simulink model "Modelo_del_sistema"  (R2018a)
settings: Solver=VariableStepAuto  StartTime=0  StopTime=2678400  FixedStep=45  RelTol=1e-3  EnableMultiTasking=on
libraries: simulink x2
(part 1 of 2)
settings Model: Creator=»Paul117x«  LastModifiedBy=Paul
settings OptimizationCC: LifeSpan=inf
settings DebuggingCC: SFUnexpectedBacktrackingDiag=warning  SFNoUnconditionalDefaultTransitionDiag=warning  SFExecutionAtInitializationDiag=none
settings CodeAppCC: StateflowObjectComments=on
settings GRTTargetCC: TargetLangStandard=C89/C90 (ANSI)  GeneratePreprocessorConditionals=Disable all
settings ConfigComp: CovMetricSettings=dw  CovHtmlReporting=on  CovSaveCumulativeToWorkspaceVar=on  CovSaveSingleToWorkspaceVar=on  CovExternalEMLEnable=off
settings SimscapeCC: SimscapeNormalizeSystem=off

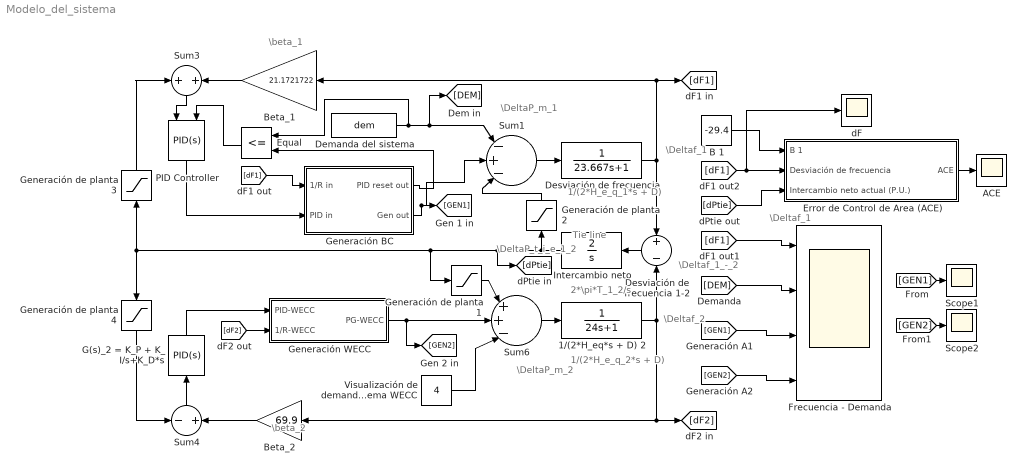
== system Modelo_del_sistema ==
  note: \Deltaf_1
  note: 2*\pi*T_1_2/s
  note: 1/(2*H_e_q_1*s + D)
  note: \beta_2
  note: \beta_1
  note: Tie line
  note: \DeltaP_m_2
  note: \Deltaf_1_-_2
  note: \DeltaP_t_i_e_1_2
  note: \Deltaf_2
  note: \Deltaf_1
  note: \DeltaP_m_1
  note: 1/(2*H_e_q_2*s + D)
  1/(2*H_eq*s + D) 2 : TransferFcn  Denominator=[24 1]
  ACE : Scope
  B 1 : Constant  Value=-29.4
  Beta_1 : Gain  Gain=21.1721722
  Beta_2 : Gain  Gain=69.9
  Demanda del sistema : FromWorkspace  VariableName=dem  SampleTime=0
  Desviación de frecuencia : TransferFcn  Denominator=[23.667 1]
  Desviación de frecuencia 1-2 : Sum  Inputs=+|-
  Equal : RelationalOperator  Operator=<=  OutDataTypeStr=boolean  RndMeth=Simplest
  Error de Control de Area (ACE) : Subsystem
  Frecuencia - Demanda : Scope  NumInputPorts=4
  G(s)_2 = K_P + K_I/s+K_D*s : simulink/Continuous/PID Controller  Controller=PID  TimeDomain=Continuous-time  SampleTime=-1  IntegratorMethod=Forward Euler  FilterMethod=Forward Euler  Form=Parallel  UseFilter=on  ControllerParametersSource=internal  P=0  I=0.00249882658784488  D=0  N=100  InitialConditionSource=internal  InitialConditionForIntegrator=0  InitialConditionForFilter=0  ExternalReset=none  LimitOutput=off  UpperSaturationLimit=inf  LowerSaturationLimit=-inf  LinearizeAsGain=on  AntiWindupMode=none  Kb=1  TrackingMode=off  Kt=1  PParamMin=[]  PParamMax=[]  IParamMin=[]  IParamMax=[]  DParamMin=[]  DParamMax=[]  NParamMin=[]  NParamMax=[]  KbParamMin=[]  KbParamMax=[]  KtParamMin=[]  KtParamMax=[]  POutMin=[]  POutMax=[]  IOutMin=[]  IOutMax=[]  DOutMin=[]  DOutMax=[]  NOutMin=[]  NOutMax=[]  KbOutMin=[]  KbOutMax=[]  KtOutMin=[]  KtOutMax=[]  IntegratorOutMin=[]  IntegratorOutMax=[]  FilterOutMin=[]  FilterOutMax=[]  SumOutMin=[]  SumOutMax=[]  SumI1OutMin=[]  SumI1OutMax=[]  SumI2OutMin=[]  SumI2OutMax=[]  SumI3OutMin=[]  SumI3OutMax=[]  SumDOutMin=[]  SumDOutMax=[]  SaturationOutMin=[]  SaturationOutMax=[]  IntegratorContinuousStateAttributes=''  IntegratorStateMustResolveToSignalObject=off  IntegratorRTWStateStorageClass=Auto  FilterContinuousStateAttributes=''  FilterStateMustResolveToSignalObject=off  FilterRTWStateStorageClass=Auto  DifferentiatorICPrevScaledInput=0  DifferentiatorOutMin=[]  DifferentiatorOutMax=[]  FilterDiffOutCoefMin=[]  FilterDiffOutCoefMax=[]  SumDenOutMin=[]  SumDenOutMax=[]  SumNumOutMin=[]  SumNumOutMax=[]  ReciprocalOutMin=[]  ReciprocalOutMax=[]  DivideOutMin=[]  DivideOutMax=[]  TunerSelectOption=Transfer Function Based (PID Tuner App)
  Generación BC : Subsystem
  Generación WECC : Subsystem
  Generación de planta 1 : Saturate  UpperLimit=0.4  LowerLimit=-0.8
  Generación de planta 2 : Saturate  UpperLimit=0.8  LowerLimit=-0.4
  Generación de planta 3 : Saturate  UpperLimit=0.8  LowerLimit=-0.4
  Generación de planta 4 : Saturate  UpperLimit=0.4  LowerLimit=-0.8
  Intercambio neto : TransferFcn  Numerator=[2]  Denominator=[1 0]
  PID Controller : simulink/Continuous/PID Controller  Controller=PID  TimeDomain=Continuous-time  SampleTime=-1  IntegratorMethod=Forward Euler  FilterMethod=Forward Euler  Form=Parallel  UseFilter=on  ControllerParametersSource=internal  P=0  I=0.00419020704903793  D=0  N=100  InitialConditionSource=internal  InitialConditionForIntegrator=0  InitialConditionForFilter=0  ExternalReset=falling  LimitOutput=on  UpperSaturationLimit=2.577  LowerSaturationLimit=-2.577  LinearizeAsGain=on  AntiWindupMode=clamping  Kb=1  TrackingMode=off  Kt=1  PParamMin=[]  PParamMax=[]  IParamMin=[]  IParamMax=[]  DParamMin=[]  DParamMax=[]  NParamMin=[]  NParamMax=[]  KbParamMin=[]  KbParamMax=[]  KtParamMin=[]  KtParamMax=[]  POutMin=[]  POutMax=[]  IOutMin=[]  IOutMax=[]  DOutMin=[]  DOutMax=[]  NOutMin=[]  NOutMax=[]  KbOutMin=[]  KbOutMax=[]  KtOutMin=[]  KtOutMax=[]  IntegratorOutMin=[]  IntegratorOutMax=[]  FilterOutMin=[]  FilterOutMax=[]  SumOutMin=[]  SumOutMax=[]  SumI1OutMin=[]  SumI1OutMax=[]  SumI2OutMin=[]  SumI2OutMax=[]  SumI3OutMin=[]  SumI3OutMax=[]  SumDOutMin=[]  SumDOutMax=[]  SaturationOutMin=[]  SaturationOutMax=[]  IntegratorContinuousStateAttributes=''  IntegratorStateMustResolveToSignalObject=off  IntegratorRTWStateStorageClass=Auto  FilterContinuousStateAttributes=''  FilterStateMustResolveToSignalObject=off  FilterRTWStateStorageClass=Auto  DifferentiatorICPrevScaledInput=0  DifferentiatorOutMin=[]  DifferentiatorOutMax=[]  FilterDiffOutCoefMin=[]  FilterDiffOutCoefMax=[]  SumDenOutMin=[]  SumDenOutMax=[]  SumNumOutMin=[]  SumNumOutMax=[]  ReciprocalOutMin=[]  ReciprocalOutMax=[]  DivideOutMin=[]  DivideOutMax=[]  TunerSelectOption=Transfer Function Based (PID Tuner App)
  Scope1 : Scope
  Scope2 : Scope
  Sum1 : Sum  Inputs=||-|+|-||
  Sum3 : Sum  Inputs=+|+
  Sum4 : Sum  Inputs=-|+
  Sum6 : Sum  Inputs=||+|+|-||
  Visualización de demanda en sistema WECC : Constant  Value=4
  dF : Scope
  wires:
  Sum1/1 -> Desviación de frecuencia/1
  1/(2*H_eq*s + D) 2/1 -> Desviación de frecuencia 1-2/2, [dF2], Beta_2/1
  Beta_1/1 -> Sum3/2
  Beta_2/1 -> Sum4/2
  Sum4/1 -> G(s)_2 = K_P + K_I/s+K_D*s/1
  B 1/1 -> Error de Control de Area (ACE)/1(B 1)
  Error de Control de Area (ACE)/1(ACE) -> ACE/1
  G(s)_2 = K_P + K_I/s+K_D*s/1 -> Generación WECC/1(PID-WECC)
  Desviación de frecuencia 1-2/1 -> Intercambio neto/1
  Sum6/1 -> 1/(2*H_eq*s + D) 2/1
  Generación WECC/1(PG-WECC) -> Sum6/2, [GEN2]
  [DEM] -> Frecuencia - Demanda/2
  Demanda del sistema/1 -> Equal/1, Sum1/1, [DEM]
  Visualización de demanda en sistema WECC/1 -> Sum6/3
  Intercambio neto/1 -> Generación de planta 1/1, Generación de planta 4/1, Generación de planta 3/1, [dPtie], Generación de planta 2/1
  Generación de planta 1/1 -> Sum6/1
  Sum3/1 -> PID Controller/1
  PID Controller/1 -> Generación BC/2(PID in)
  Equal/1 -> PID Controller/2
  [dF1] -> Generación BC/1(1/R in)
  Generación BC/1(PID reset out) -> Equal/2
  Generación BC/2(Gen out) -> Sum1/2, [GEN1]
  [dF1] -> Frecuencia - Demanda/1
  [dF2] -> Generación WECC/2(1/R-WECC)
  [dPtie] -> Error de Control de Area (ACE)/3(Intercambio neto actual (P.U.))
  Desviación de frecuencia/1 -> [dF1], Beta_1/1, Desviación de frecuencia 1-2/1
  [GEN2] -> Frecuencia - Demanda/4
  [GEN1] -> Frecuencia - Demanda/3
  [dF1] -> dF/1, Error de Control de Area (ACE)/2(Desviación de frecuencia)
  [GEN1] -> Scope1/1
  [GEN2] -> Scope2/1
  Generación de planta 2/1 -> Sum1/3
  Generación de planta 3/1 -> Sum3/1
  Generación de planta 4/1 -> Sum4/1

== system Modelo_del_sistema/Error de Control de Area (ACE) ==
  note: \Deltaf_1
  note: Conversión de frecuencia
      | 	     P.U. a Hz.
  note: 10*B_i*(\Deltaf)
  note: IN_a - IN_p
  note: Conversión de intercambio
      | 	     P.U. a MW.
  B 1 : Inport
  Desviación de frecuencia : Inport  Port=2
  Intercambio neto actual (P.U.) : Inport  Port=3
  Constante : Constant  Value=10
  Hz Base : Constant  Value=60
  Intercambio programado (MW) : Constant  Value=0
  MW Base : Constant  Value=1000
  Product{,1..3} (4 alike) : Product  Inputs=**
  Sum7 : Sum  Inputs=+|-
  Sum9 : Sum  Inputs=-|+
  ACE : Outport
  wires:
  B 1/1 -> Product2/2
  Hz Base/1 -> Product/2
  Product/1 -> Product1/1
  MW Base/1 -> Product3/2
  Sum9/1 -> ACE/1
  Constante/1 -> Product1/2
  Product2/1 -> Sum9/1
  Sum7/1 -> Sum9/2
  Desviación de frecuencia/1 -> Product/1
  Intercambio neto actual (P.U.)/1 -> Product3/1
  Product3/1 -> Sum7/1
  Intercambio programado (MW)/1 -> Sum7/2
  Product1/1 -> Product2/1

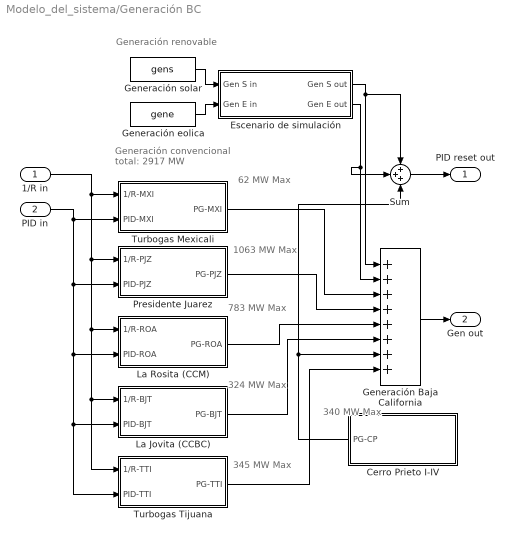
== system Modelo_del_sistema/Generación BC ==
  note: Generación renovable
  note: Generación convencional
      | 	 total: 2917 MW
  note: 62 MW
      |   Max
  note: 1063 MW
      |     Max
  note: 783 MW
      |    Max
  note: 324 MW
      |    Max
  note: 340 MW
      |   Max
  note: 345 MW
      |    Max
  1/R in : Inport
  PID in : Inport  Port=2
  Cerro Prieto I-IV : Subsystem
  Escenario de simulación : Subsystem
  Generación Baja California : Sum  Inputs=+||+||+||+||+||+||+||+
  Generación eolica : FromWorkspace  VariableName=gene  SampleTime=0
  Generación solar : FromWorkspace  VariableName=gens  SampleTime=0
  La Jovita (CCBC) : Subsystem
  La Rosita (CCM) : Subsystem
  Presidente Juarez : Subsystem
  Sum : Sum  Inputs=3
  Turbogas Mexicali : Subsystem
  Turbogas Tijuana : Subsystem
  PID reset out : Outport
  Gen out : Outport  Port=2
  wires:
  La Jovita (CCBC)/1(PG-BJT) -> Generación Baja California/6
  Generación solar/1 -> Escenario de simulación/1(Gen S in)
  PID in/1 -> Turbogas Mexicali/2(PID-MXI), Presidente Juarez/2(PID-PJZ), La Rosita (CCM)/2(PID-ROA), La Jovita (CCBC)/2(PID-BJT), Turbogas Tijuana/2(PID-TTI)
  Escenario de simulación/2(Gen E out) -> Sum/2, Generación Baja California/2
  1/R in/1 -> Turbogas Mexicali/1(1/R-MXI), Presidente Juarez/1(1/R-PJZ), La Rosita (CCM)/1(1/R-ROA), La Jovita (CCBC)/1(1/R-BJT), Turbogas Tijuana/1(1/R-TTI)
  Escenario de simulación/1(Gen S out) -> Sum/1, Generación Baja California/1
  Cerro Prieto I-IV/1(PG-CP) -> Sum/3, Generación Baja California/7
  Presidente Juarez/1(PG-PJZ) -> Generación Baja California/4
  Generación eolica/1 -> Escenario de simulación/2(Gen E in)
  Turbogas Mexicali/1(PG-MXI) -> Generación Baja California/3
  Turbogas Tijuana/1(PG-TTI) -> Generación Baja California/8
  Generación Baja California/1 -> Gen out/1
  La Rosita (CCM)/1(PG-ROA) -> Generación Baja California/5
  Sum/1 -> PID reset out/1

== system Modelo_del_sistema/Generación WECC ==
  PID-WECC : Inport
  1/R-WECC : Inport  Port=2
  1/(sT_g + 1) 2 : TransferFcn  Denominator=[0.04 1]
  1/R2 : Gain  Gain=20
  Generación extra área 2 : TransferFcn  Denominator=[0.2 1]
  Sum5 : Sum  Inputs=|--
  PG-WECC : Outport
  wires:
  1/R2/1 -> Sum5/2
  PID-WECC/1 -> Sum5/1
  1/R-WECC/1 -> 1/R2/1
  1/(sT_g + 1) 2/1 -> Generación extra área 2/1
  Sum5/1 -> 1/(sT_g + 1) 2/1
  Generación extra área 2/1 -> PG-WECC/1

== system Modelo_del_sistema/Generación BC/Cerro Prieto I-IV ==
  note: Heq = 4.593
  CP Gen : Constant  Value=0.34
  PG-CP : Outport
  wires:
  CP Gen/1 -> PG-CP/1

== system Modelo_del_sistema/Generación BC/Escenario de simulación ==
  Gen S in : Inport
  Gen E in : Inport  Port=2
  Constant : Constant  Value=0
  Eólico Ago : Subsystem
  Eólico Dic : Subsystem
  Multiport Switch : MultiPortSwitch  Inputs=2  DataPortForDefault=Additional data port
  Multiport Switch2 : MultiPortSwitch  Inputs=2  DataPortForDefault=Additional data port
  Scope : Scope
  Selector : FromWorkspace  VariableName=p  OutDataTypeStr=double  SampleTime=0  OutputAfterFinalValue=Holding final value
  Solar Ago : Subsystem
  Solar Dic : Subsystem
  Gen S out : Outport
  Gen E out : Outport  Port=2
  wires:
  Gen E in/1 -> Eólico Ago/1(Gen E in), Eólico Dic/1(Gen E in)
  Eólico Ago/1(Gen E out) -> Multiport Switch2/2
  Eólico Dic/1(Gen E out) -> Multiport Switch2/3
  Multiport Switch2/1 -> Scope/1, Gen E out/1
  Multiport Switch/1 -> Gen S out/1
  Selector/1 -> Multiport Switch/1, Multiport Switch2/1
  Constant/1 -> Multiport Switch2/4, Multiport Switch/4
  Solar Dic/1(Gen S out) -> Multiport Switch/3
  Solar Ago/1(Gen S out) -> Multiport Switch/2
  Gen S in/1 -> Solar Dic/1(Gen S in), Solar Ago/1(Gen S in)

== system Modelo_del_sistema/Generación BC/La Jovita (CCBC) ==
  note: Heq = 4.2
  1/R-BJT : Inport
  PID-BJT : Inport  Port=2
  1/(sT_g + 1)1 : TransferFcn  Denominator=[2.675 1]
  1/(sT_t + 1)1 : TransferFcn  Denominator=[0.71 1]
  1/R2 : Gain  Gain=16.50615303
  Saturation : Saturate  UpperLimit=0.324  LowerLimit=0
  Sum1 : Sum  Inputs=--|
  PG-BJT : Outport
  wires:
  1/(sT_g + 1)1/1 -> 1/(sT_t + 1)1/1
  Sum1/1 -> 1/(sT_g + 1)1/1
  1/R-BJT/1 -> 1/R2/1
  1/R2/1 -> Sum1/1
  1/(sT_t + 1)1/1 -> Saturation/1
  Saturation/1 -> PG-BJT/1
  PID-BJT/1 -> Sum1/2

== system Modelo_del_sistema/Generación BC/La Rosita (CCM) ==
  note: T2 = 0.2
  note: 1/R = 24.85720114
  note: T_1 = 1
  note: Heq = 5.893
  1/R-ROA : Inport
  PID-ROA : Inport  Port=2
  1/(sT_g + 1)1 : TransferFcn  Denominator=[0.15 1]
  1/(sT_t + 1)1 : TransferFcn  Denominator=[0.05 1]
  1/R1 : Gain  Gain=24.85720114
  Saturation : Saturate  UpperLimit=0.783  LowerLimit=0
  Sum1 : Sum  Inputs=--|
  PG-ROA : Outport
  wires:
  1/(sT_g + 1)1/1 -> 1/(sT_t + 1)1/1
  Sum1/1 -> 1/(sT_g + 1)1/1
  1/R-ROA/1 -> 1/R1/1
  1/R1/1 -> Sum1/1
  1/(sT_t + 1)1/1 -> Saturation/1
  Saturation/1 -> PG-ROA/1
  PID-ROA/1 -> Sum1/2

== system Modelo_del_sistema/Generación BC/Presidente Juarez ==
  note: T2 = 1.56
  note: T1 = 2.032
  note: Heq = 3.38
  1/R-PJZ : Inport
  PID-PJZ : Inport  Port=2
  1/(sT_g + 1)1 : TransferFcn  Denominator=[0.2 1]
  1/(sT_t + 1)1 : TransferFcn  Denominator=[0.1 1]
  1/R1 : Gain  Gain=18.56344588
  Saturation : Saturate  UpperLimit=1.063  LowerLimit=0
  Sum1 : Sum  Inputs=--|
  PG-PJZ : Outport
  wires:
  1/(sT_g + 1)1/1 -> 1/(sT_t + 1)1/1
  Sum1/1 -> 1/(sT_g + 1)1/1
  1/R1/1 -> Sum1/1
  1/R-PJZ/1 -> 1/R1/1
  1/(sT_t + 1)1/1 -> Saturation/1
  Saturation/1 -> PG-PJZ/1
  PID-PJZ/1 -> Sum1/2

== system Modelo_del_sistema/Generación BC/Turbogas Mexicali ==
  note: 62 MW de generación MAX
  note: Heq = 3.666
  1/R-MXI : Inport
  PID-MXI : Inport  Port=2
  1/(sT_g + 1) : TransferFcn  Denominator=[0.16666 1]
  1/(sT_t + 1) : TransferFcn  Denominator=[0.366666 1]
  1/R1 : Gain  Gain=19.09999982
  Saturation : Saturate  UpperLimit=0.062  LowerLimit=0
  Sum : Sum  Inputs=--|
  PG-MXI : Outport
  wires:
  1/(sT_g + 1)/1 -> 1/(sT_t + 1)/1
  Sum/1 -> 1/(sT_g + 1)/1
  1/R-MXI/1 -> 1/R1/1
  1/R1/1 -> Sum/1
  1/(sT_t + 1)/1 -> Saturation/1
  Saturation/1 -> PG-MXI/1
  PID-MXI/1 -> Sum/2

== system Modelo_del_sistema/Generación BC/Turbogas Tijuana ==
  note: Heq = 5.91
  1/R-TTI : Inport
  PID-TTI : Inport  Port=2
  1/(sT_g + 1)1 : TransferFcn  Denominator=[0.1 1]
  1/(sT_t + 1)1 : TransferFcn  Denominator=[0.2 1]
  1/R1 : Gain  Gain=21.83406114
  Saturation : Saturate  UpperLimit=0.345  LowerLimit=0
  Sum1 : Sum  Inputs=--|
  PG-TTI : Outport
  wires:
  1/(sT_g + 1)1/1 -> 1/(sT_t + 1)1/1
  Sum1/1 -> 1/(sT_g + 1)1/1
  1/R1/1 -> Sum1/1
  1/R-TTI/1 -> 1/R1/1
  1/(sT_t + 1)1/1 -> Saturation/1
  Saturation/1 -> PG-TTI/1
  PID-TTI/1 -> Sum1/2

== system Modelo_del_sistema/Generación BC/Escenario de simulación/Eólico Ago ==
  Gen E in : Inport
  Falla día 13 : Subsystem
  Falla día 16 : Subsystem
  Falla día 18 : Subsystem
  Falla día 21 : Subsystem
  Falla día 25 : Subsystem
  Falla día 28 : Subsystem
  Falla día 30 : Subsystem
  Falla día 6 : Subsystem
  Falla día 8 : Subsystem
  Gen E out : Outport
  wires:
  Gen E in/1 -> Falla día 6/1(In1)
  Falla día 16/1(Out1) -> Falla día 18/1(In1)
  Falla día 25/1(Out1) -> Falla día 28/1(In1)
  Falla día 28/1(Out1) -> Falla día 30/1(In1)
  Falla día 13/1(Out1) -> Falla día 16/1(In1)
  Falla día 21/1(Out1) -> Falla día 25/1(In1)
  Falla día 30/1(Out1) -> Gen E out/1
  Falla día 18/1(Out1) -> Falla día 21/1(In1)
  Falla día 8/1(Out1) -> Falla día 13/1(In1)
  Falla día 6/1(Out1) -> Falla día 8/1(In1)

== system Modelo_del_sistema/Generación BC/Escenario de simulación/Eólico Dic ==
  Gen E in : Inport
  Falla día 12 : Subsystem
  Falla día 14 : Subsystem
  Falla día 16 : Subsystem
  Falla día 20 : Subsystem
  Falla día 24 : Subsystem
  Falla día 30 : Subsystem
  Falla día 4 : Subsystem
  Falla día 8 : Subsystem
  Falla día 9 : Subsystem
  Gen E out : Outport
  wires:
  Gen E in/1 -> Falla día 4/1(In1)
  Falla día 4/1(Out1) -> Falla día 8/1(In1)
  Falla día 8/1(Out1) -> Falla día 9/1(In1)
  Falla día 9/1(Out1) -> Falla día 12/1(In1)
  Falla día 12/1(Out1) -> Falla día 14/1(In1)
  Falla día 14/1(Out1) -> Falla día 16/1(In1)
  Falla día 16/1(Out1) -> Falla día 20/1(In1)
  Falla día 20/1(Out1) -> Falla día 24/1(In1)
  Falla día 24/1(Out1) -> Falla día 30/1(In1)
  Falla día 30/1(Out1) -> Gen E out/1

== system Modelo_del_sistema/Generación BC/Escenario de simulación/Solar Ago ==
  Gen S in : Inport
  Falla día 12 : Subsystem
  Falla día 16 : Subsystem
  Falla día 18 : Subsystem
  Falla día 20 : Subsystem
  Falla día 25 : Subsystem
  Falla día 26 : Subsystem
  Falla día 28 : Subsystem
  Falla día 5 : Subsystem
  Falla día 9 : Subsystem
  Gen S out : Outport
  wires:
  Falla día 5/1(Out1) -> Falla día 9/1(In1)
  Falla día 9/1(Out1) -> Falla día 12/1(In1)
  Gen S in/1 -> Falla día 5/1(In1)
  Falla día 20/1(Out1) -> Falla día 25/1(In1)
  Falla día 25/1(Out1) -> Falla día 26/1(In1)
  Falla día 26/1(Out1) -> Falla día 28/1(In1)
  Falla día 12/1(Out1) -> Falla día 16/1(In1)
  Falla día 28/1(Out1) -> Gen S out/1
  Falla día 18/1(Out1) -> Falla día 20/1(In1)
  Falla día 16/1(Out1) -> Falla día 18/1(In1)

== system Modelo_del_sistema/Generación BC/Escenario de simulación/Solar Dic ==
  Gen S in : Inport
  Falla día 13 : Subsystem
  Falla día 16 : Subsystem
  Falla día 2 : Subsystem
  Falla día 21 : Subsystem
  Falla día 23 : Subsystem
  Falla día 24 : Subsystem
  Falla día 28 : Subsystem
  Falla día 30 : Subsystem
  Falla día 4 : Subsystem
  Gen S out : Outport
  wires:
  Gen S in/1 -> Falla día 2/1(In1)
  Falla día 4/1(Out1) -> Falla día 13/1(In1)
  Falla día 2/1(Out1) -> Falla día 4/1(In1)
  Falla día 13/1(Out1) -> Falla día 16/1(In1)
  Falla día 16/1(Out1) -> Falla día 21/1(In1)
  Falla día 23/1(Out1) -> Falla día 24/1(In1)
  Falla día 21/1(Out1) -> Falla día 23/1(In1)
  Falla día 24/1(Out1) -> Falla día 28/1(In1)
  Falla día 28/1(Out1) -> Falla día 30/1(In1)
  Falla día 30/1(Out1) -> Gen S out/1

== system Modelo_del_sistema/Generación BC/Escenario de simulación/Eólico Ago/Falla día 13 ==
  In1 : Inport
  Add : Sum
  Clock : Clock
  Clock1 : Clock
  Product : Product
  Sine Wave : Sin  Amplitude=0.73  Frequency=0.00086071/2  Phase=pi/2+pi/4.5  SampleTime=0
  Switch : Switch  Threshold=1097000
  Switch1 : Switch  Threshold=1104300
  Out1 : Outport
  wires:
  Add/1 -> Switch/1
  Product/1 -> Add/2
  Clock/1 -> Switch/2
  In1/1 -> Switch/3, Product/1, Add/1, Switch1/1
  Switch1/1 -> Out1/1
  Sine Wave/1 -> Product/2
  Clock1/1 -> Switch1/2
  Switch/1 -> Switch1/3

== system Modelo_del_sistema/Generación BC/Escenario de simulación/Eólico Ago/Falla día 16 ==
  In1 : Inport
  Add : Sum
  Clock : Clock
  Clock1 : Clock
  Product : Product
  Sine Wave : Sin  Amplitude=0.20  Frequency=0.000455303  Phase=3*pi/2+pi+pi/8.1  SampleTime=0
  Switch : Switch  Threshold=1355000
  Switch1 : Switch  Threshold=1361900
  Out1 : Outport
  wires:
  Add/1 -> Switch/1
  Product/1 -> Add/2
  Clock/1 -> Switch/2
  In1/1 -> Switch/3, Product/1, Add/1, Switch1/1
  Switch1/1 -> Out1/1
  Sine Wave/1 -> Product/2
  Clock1/1 -> Switch1/2
  Switch/1 -> Switch1/3

== system Modelo_del_sistema/Generación BC/Escenario de simulación/Eólico Ago/Falla día 18 ==
  In1 : Inport
  Add : Sum
  Clock : Clock
  Clock1 : Clock
  Product : Product
  Sine Wave : Sin  Amplitude=0.71  Frequency=0.000263999  Phase=pi/4+pi/93  SampleTime=0
  Switch : Switch  Threshold=1532000
  Switch1 : Switch  Threshold=1543900
  Out1 : Outport
  wires:
  Add/1 -> Switch/1
  Product/1 -> Add/2
  Clock/1 -> Switch/2
  In1/1 -> Switch/3, Product/1, Add/1, Switch1/1
  Switch1/1 -> Out1/1
  Sine Wave/1 -> Product/2
  Clock1/1 -> Switch1/2
  Switch/1 -> Switch1/3

== system Modelo_del_sistema/Generación BC/Escenario de simulación/Eólico Ago/Falla día 21 ==
  In1 : Inport
  Add : Sum
  Clock : Clock
  Clock1 : Clock
  Product : Product
  Sine Wave : Sin  Amplitude=0.54  Frequency=0.000213714  Phase=-pi/4-pi/16  SampleTime=0
  Switch : Switch  Threshold=1783300
  Switch1 : Switch  Threshold=1798000
  Out1 : Outport
  wires:
  Add/1 -> Switch/1
  Product/1 -> Add/2
  Clock/1 -> Switch/2
  In1/1 -> Switch/3, Product/1, Add/1, Switch1/1
  Switch1/1 -> Out1/1
  Sine Wave/1 -> Product/2
  Clock1/1 -> Switch1/2
  Switch/1 -> Switch1/3

== system Modelo_del_sistema/Generación BC/Escenario de simulación/Eólico Ago/Falla día 25 ==
  In1 : Inport
  Add : Sum
  Clock : Clock
  Clock1 : Clock
  Product : Product
  Sine Wave : Sin  Amplitude=0.44  Frequency=0.000259636  Phase=pi-pi/4.33  SampleTime=0
  Switch : Switch  Threshold=2132400
  Switch1 : Switch  Threshold=2144500
  Out1 : Outport
  wires:
  Add/1 -> Switch/1
  Product/1 -> Add/2
  Clock/1 -> Switch/2
  In1/1 -> Switch/3, Product/1, Add/1, Switch1/1
  Switch1/1 -> Out1/1
  Sine Wave/1 -> Product/2
  Clock1/1 -> Switch1/2
  Switch/1 -> Switch1/3

== system Modelo_del_sistema/Generación BC/Escenario de simulación/Eólico Ago/Falla día 28 ==
  In1 : Inport
  Add : Sum
  Clock : Clock
  Clock1 : Clock
  Product : Product
  Sine Wave : Sin  Amplitude=0.95  Frequency=0.000255414  Phase=-pi/3.001  SampleTime=0
  Switch : Switch  Threshold=2402600
  Switch1 : Switch  Threshold=2414900
  Out1 : Outport
  wires:
  Add/1 -> Switch/1
  Product/1 -> Add/2
  Clock/1 -> Switch/2
  In1/1 -> Switch/3, Product/1, Add/1, Switch1/1
  Switch1/1 -> Out1/1
  Sine Wave/1 -> Product/2
  Clock1/1 -> Switch1/2
  Switch/1 -> Switch1/3

== system Modelo_del_sistema/Generación BC/Escenario de simulación/Eólico Ago/Falla día 30 ==
  In1 : Inport
  Add : Sum
  Clock : Clock
  Clock1 : Clock
  Product : Product
  Sine Wave : Sin  Amplitude=0.93  Frequency=0.000119000  Phase=-pi/32.76  SampleTime=0
  Switch : Switch  Threshold=2561600
  Switch1 : Switch  Threshold=2588000
  Out1 : Outport
  wires:
  Add/1 -> Switch/1
  Product/1 -> Add/2
  Clock/1 -> Switch/2
  In1/1 -> Switch/3, Product/1, Add/1, Switch1/1
  Switch1/1 -> Out1/1
  Sine Wave/1 -> Product/2
  Clock1/1 -> Switch1/2
  Switch/1 -> Switch1/3

== system Modelo_del_sistema/Generación BC/Escenario de simulación/Eólico Ago/Falla día 6 ==
  In1 : Inport
  Add : Sum
  Clock : Clock
  Clock1 : Clock
  Product : Product
  Scope : Scope  NumInputPorts=2
  Sine Wave : Sin  Amplitude=0.52  Frequency=0.000213714  Phase=pi/2+pi+pi/42  SampleTime=0
  Switch : Switch  Threshold=492100
  Switch1 : Switch  Threshold=506800
  Out1 : Outport
  wires:
  Add/1 -> Switch/1
  Product/1 -> Add/2
  Clock/1 -> Switch/2
  In1/1 -> Scope/1, Switch/3, Product/1, Add/1, Switch1/1
  Switch1/1 -> Scope/2, Out1/1
  Sine Wave/1 -> Product/2
  Clock1/1 -> Switch1/2
  Switch/1 -> Switch1/3

== system Modelo_del_sistema/Generación BC/Escenario de simulación/Eólico Ago/Falla día 8 ==
  In1 : Inport
  Add : Sum
  Clock : Clock
  Clock1 : Clock
  Product : Product
  Sine Wave : Sin  Amplitude=0.62  Frequency=3.779359583e-4/2  Phase=-pi/2-pi/24  SampleTime=0
  Switch : Switch  Threshold=657450
  Switch1 : Switch  Threshold=674075
  Out1 : Outport
  wires:
  Add/1 -> Switch/1
  Product/1 -> Add/2
  Clock/1 -> Switch/2
  In1/1 -> Switch/3, Product/1, Add/1, Switch1/1
  Switch1/1 -> Out1/1
  Sine Wave/1 -> Product/2
  Clock1/1 -> Switch1/2
  Switch/1 -> Switch1/3

== system Modelo_del_sistema/Generación BC/Escenario de simulación/Eólico Dic/Falla día 12 ==
  In1 : Inport
  Add : Sum
  Clock : Clock
  Clock1 : Clock
  Product : Product
  Sine Wave : Sin  Amplitude=0.94  Frequency=0.000475999  Phase=pi-pi/3.66  SampleTime=0
  Switch : Switch  Threshold=991800
  Switch1 : Switch  Threshold=998400
  Out1 : Outport
  wires:
  Add/1 -> Switch/1
  Product/1 -> Add/2
  Clock/1 -> Switch/2
  In1/1 -> Product/1, Add/1, Switch1/1, Switch/3
  Switch1/1 -> Out1/1
  Sine Wave/1 -> Product/2
  Clock1/1 -> Switch1/2
  Switch/1 -> Switch1/3

== system Modelo_del_sistema/Generación BC/Escenario de simulación/Eólico Dic/Falla día 14 ==
  In1 : Inport
  Add : Sum
  Clock : Clock
  Clock1 : Clock
  Product : Product
  Sine Wave : Sin  Amplitude=0.20  Frequency=0.000180551  Phase=-3*pi/4-pi/23.5  SampleTime=0
  Switch : Switch  Threshold=1179600
  Switch1 : Switch  Threshold=1197000
  Out1 : Outport
  wires:
  Add/1 -> Switch/1
  Product/1 -> Add/2
  Clock/1 -> Switch/2
  In1/1 -> Product/1, Add/1, Switch1/1, Switch/3
  Switch1/1 -> Out1/1
  Sine Wave/1 -> Product/2
  Clock1/1 -> Switch1/2
  Switch/1 -> Switch1/3

== system Modelo_del_sistema/Generación BC/Escenario de simulación/Eólico Dic/Falla día 16 ==
  In1 : Inport
  Add : Sum
  Clock : Clock
  Clock1 : Clock
  Product : Product
  Sine Wave : Sin  Amplitude=0.41  Frequency=0.000515015  Phase=-pi/2-pi/128  SampleTime=0
  Switch : Switch  Threshold=1326800
  Switch1 : Switch  Threshold=1332900
  Out1 : Outport
  wires:
  Add/1 -> Switch/1
  Product/1 -> Add/2
  Clock/1 -> Switch/2
  In1/1 -> Switch/3, Product/1, Add/1, Switch1/1
  Switch1/1 -> Out1/1
  Sine Wave/1 -> Product/2
  Clock1/1 -> Switch1/2
  Switch/1 -> Switch1/3

== system Modelo_del_sistema/Generación BC/Escenario de simulación/Eólico Dic/Falla día 20 ==
  In1 : Inport
  Add : Sum
  Clock : Clock
  Clock1 : Clock
  Product : Product
  Sine Wave : Sin  Amplitude=0.36  Frequency=0.000356999  Phase=-pi/2-pi/10  SampleTime=0
  Switch : Switch  Threshold=1686100
  Switch1 : Switch  Threshold=1694900
  Out1 : Outport
  wires:
  Add/1 -> Switch/1
  Product/1 -> Add/2
  Clock/1 -> Switch/2
  In1/1 -> Switch/3, Product/1, Add/1, Switch1/1
  Switch1/1 -> Out1/1
  Sine Wave/1 -> Product/2
  Clock1/1 -> Switch1/2
  Switch/1 -> Switch1/3

== system Modelo_del_sistema/Generación BC/Escenario de simulación/Eólico Dic/Falla día 24 ==
  In1 : Inport
  Add : Sum
  Clock : Clock
  Clock1 : Clock
  Product : Product
  Sine Wave : Sin  Amplitude=0.59  Frequency=0.000345230  Phase=pi-pi/10.1  SampleTime=0
  Switch : Switch  Threshold=2002900
  Switch1 : Switch  Threshold=2012000
  Out1 : Outport
  wires:
  Add/1 -> Switch/1
  Product/1 -> Add/2
  Clock/1 -> Switch/2
  In1/1 -> Switch/3, Product/1, Add/1, Switch1/1
  Switch1/1 -> Out1/1
  Sine Wave/1 -> Product/2
  Clock1/1 -> Switch1/2
  Switch/1 -> Switch1/3

== system Modelo_del_sistema/Generación BC/Escenario de simulación/Eólico Dic/Falla día 30 ==
  In1 : Inport
  Add : Sum
  Clock : Clock
  Clock1 : Clock
  Product : Product
  Sine Wave : Sin  Amplitude=0.3  Frequency=0.000073060  Phase=pi/2+pi/10.21  SampleTime=0
  Switch : Switch  Threshold=2511300
  Switch1 : Switch  Threshold=2554300
  Out1 : Outport
  wires:
  Add/1 -> Switch/1
  Product/1 -> Add/2
  Clock/1 -> Switch/2
  In1/1 -> Switch/3, Product/1, Add/1, Switch1/1
  Switch1/1 -> Out1/1
  Sine Wave/1 -> Product/2
  Clock1/1 -> Switch1/2
  Switch/1 -> Switch1/3

== system Modelo_del_sistema/Generación BC/Escenario de simulación/Eólico Dic/Falla día 4 ==
  In1 : Inport
  Add : Sum
  Clock : Clock
  Clock1 : Clock
  Product : Product
  Sine Wave : Sin  Amplitude=0.6  Frequency=2.992e-4  Phase=-pi/2-pi/4-pi/46.5  SampleTime=0
  Switch : Switch  Threshold=312600
  Switch1 : Switch  Threshold=323100
  Out1 : Outport
  wires:
  Add/1 -> Switch/1
  Product/1 -> Add/2
  Clock/1 -> Switch/2
  In1/1 -> Switch/3, Product/1, Add/1, Switch1/1
  Switch1/1 -> Out1/1
  Sine Wave/1 -> Product/2
  Clock1/1 -> Switch1/2
  Switch/1 -> Switch1/3

== system Modelo_del_sistema/Generación BC/Escenario de simulación/Eólico Dic/Falla día 8 ==
  In1 : Inport
  Add : Sum
  Clock : Clock
  Clock1 : Clock
  Product : Product
  Sine Wave : Sin  Amplitude=0.41  Frequency=0.000951998  Phase=-pi/1.57  SampleTime=0
  Switch : Switch  Threshold=632400
  Switch1 : Switch  Threshold=635700
  Out1 : Outport
  wires:
  Add/1 -> Switch/1
  Product/1 -> Add/2
  Clock/1 -> Switch/2
  In1/1 -> Switch/3, Product/1, Add/1, Switch1/1
  Switch1/1 -> Out1/1
  Sine Wave/1 -> Product/2
  Clock1/1 -> Switch1/2
  Switch/1 -> Switch1/3

== system Modelo_del_sistema/Generación BC/Escenario de simulación/Eólico Dic/Falla día 9 ==
  In1 : Inport
  Add : Sum
  Clock : Clock
  Clock1 : Clock
  Product : Product
  Sine Wave : Sin  Amplitude=0.21  Frequency=0.000448799  Phase=-pi-pi/3.69  SampleTime=0
  Switch : Switch  Threshold=743900
  Switch1 : Switch  Threshold=750900
  Out1 : Outport
  wires:
  Add/1 -> Switch/1
  Product/1 -> Add/2
  Clock/1 -> Switch/2
  In1/1 -> Product/1, Add/1, Switch1/1, Switch/3
  Switch1/1 -> Out1/1
  Sine Wave/1 -> Product/2
  Clock1/1 -> Switch1/2
  Switch/1 -> Switch1/3

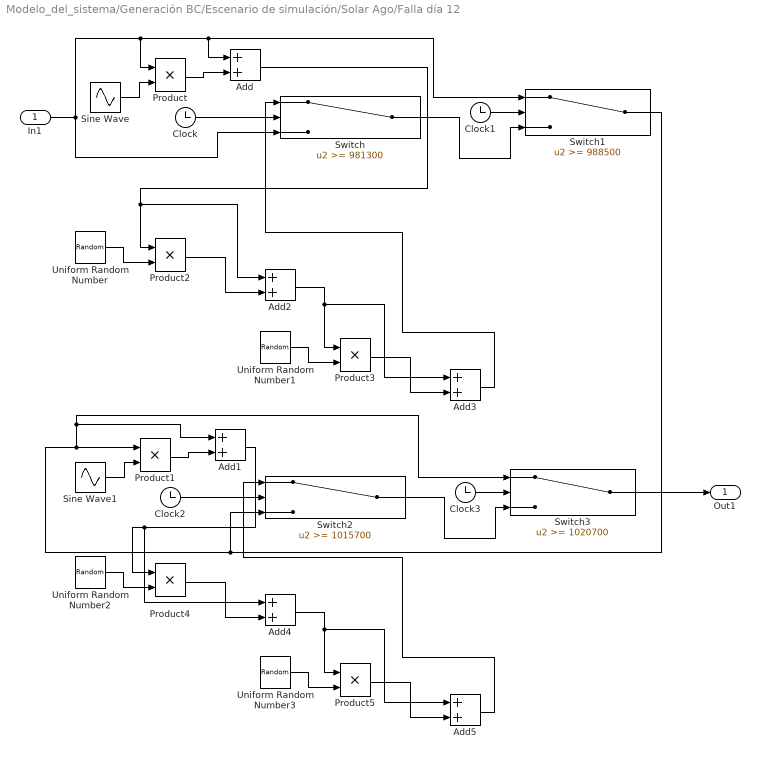
== system Modelo_del_sistema/Generación BC/Escenario de simulación/Solar Ago/Falla día 12 ==
  In1 : Inport
  Add{,1..5} (6 alike) : Sum
  Clock{,1..3} (4 alike) : Clock
  Product{,1..5} (6 alike) : Product
  Sine Wave : Sin  Amplitude=0.27  Frequency=0.000436332  Phase=pi-pi/3.4299  SampleTime=0
  Sine Wave1 : Sin  Amplitude=0.56  Frequency=0.000628319  Phase=-pi/8-pi/67  SampleTime=0
  Switch : Switch  Threshold=981300
  Switch1 : Switch  Threshold=988500
  Switch2 : Switch  Threshold=1015700
  Switch3 : Switch  Threshold=1020700
  Uniform Random Number : UniformRandomNumber  Minimum=-0.5  Maximum=0  Seed=1337  SampleTime=50
  Uniform Random Number1 : UniformRandomNumber  Minimum=-0.25  Maximum=0  Seed=69420  SampleTime=25
  Uniform Random Number2 : UniformRandomNumber  Minimum=-0.5  Maximum=0  Seed=1337  SampleTime=50
  Uniform Random Number3 : UniformRandomNumber  Minimum=-0.25  Maximum=0  Seed=69420  SampleTime=25
  Out1 : Outport
  wires:
  Product/1 -> Add/2
  Clock/1 -> Switch/2
  Sine Wave/1 -> Product/2
  Clock1/1 -> Switch1/2
  Switch/1 -> Switch1/3
  In1/1 -> Switch/3, Product/1, Add/1, Switch1/1
  Product1/1 -> Add1/2
  Clock2/1 -> Switch2/2
  Sine Wave1/1 -> Product1/2
  Clock3/1 -> Switch3/2
  Switch2/1 -> Switch3/3
  Switch3/1 -> Out1/1
  Switch1/1 -> Switch3/1, Add1/1, Product1/1, Switch2/3
  Add2/1 -> Add3/1, Product3/1
  Product3/1 -> Add3/2
  Add3/1 -> Switch/1
  Uniform Random Number1/1 -> Product3/2
  Add/1 -> Add2/1, Product2/1
  Uniform Random Number/1 -> Product2/2
  Product2/1 -> Add2/2
  Add4/1 -> Add5/1, Product5/1
  Product5/1 -> Add5/2
  Add5/1 -> Switch2/1
  Uniform Random Number3/1 -> Product5/2
  Add1/1 -> Add4/1, Product4/1
  Uniform Random Number2/1 -> Product4/2
  Product4/1 -> Add4/2

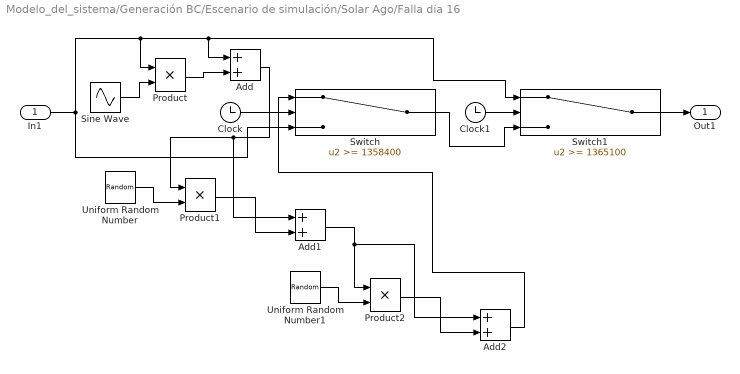
== system Modelo_del_sistema/Generación BC/Escenario de simulación/Solar Ago/Falla día 16 ==
  In1 : Inport
  Add : Sum
  Add1 : Sum
  Add2 : Sum
  Clock : Clock
  Clock1 : Clock
  Product : Product
  Product1 : Product
  Product2 : Product
  Sine Wave : Sin  Amplitude=0.70  Frequency=0.000468894  Phase=-pi/2-pi/6+pi-pi/12.6  SampleTime=0
  Switch : Switch  Threshold=1358400
  Switch1 : Switch  Threshold=1365100
  Uniform Random Number : UniformRandomNumber  Minimum=-0.5  Maximum=0  Seed=1337  SampleTime=50
  Uniform Random Number1 : UniformRandomNumber  Minimum=-0.25  Maximum=0  Seed=69420  SampleTime=25
  Out1 : Outport
  wires:
  Product/1 -> Add/2
  Clock/1 -> Switch/2
  In1/1 -> Switch/3, Product/1, Add/1, Switch1/1
  Switch1/1 -> Out1/1
  Sine Wave/1 -> Product/2
  Clock1/1 -> Switch1/2
  Switch/1 -> Switch1/3
  Add1/1 -> Add2/1, Product2/1
  Product2/1 -> Add2/2
  Add2/1 -> Switch/1
  Uniform Random Number1/1 -> Product2/2
  Add/1 -> Add1/1, Product1/1
  Uniform Random Number/1 -> Product1/2
  Product1/1 -> Add1/2

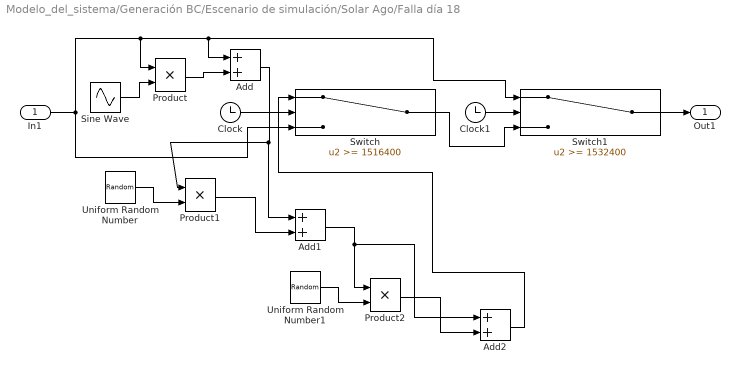
== system Modelo_del_sistema/Generación BC/Escenario de simulación/Solar Ago/Falla día 18 ==
  In1 : Inport
  Add : Sum
  Add1 : Sum
  Add2 : Sum
  Clock : Clock
  Clock1 : Clock
  Product : Product
  Product1 : Product
  Product2 : Product
  Sine Wave : Sin  Amplitude=0.29  Frequency=0.000196350  Phase=pi/4-pi/40  SampleTime=0
  Switch : Switch  Threshold=1516400
  Switch1 : Switch  Threshold=1532400
  Uniform Random Number : UniformRandomNumber  Minimum=-0.5  Maximum=0  Seed=1337  SampleTime=50
  Uniform Random Number1 : UniformRandomNumber  Minimum=-0.25  Maximum=0  Seed=69420  SampleTime=25
  Out1 : Outport
  wires:
  Product/1 -> Add/2
  Clock/1 -> Switch/2
  In1/1 -> Switch/3, Product/1, Add/1, Switch1/1
  Switch1/1 -> Out1/1
  Sine Wave/1 -> Product/2
  Clock1/1 -> Switch1/2
  Switch/1 -> Switch1/3
  Add1/1 -> Add2/1, Product2/1
  Add/1 -> Add1/1, Product1/1
  Product2/1 -> Add2/2
  Add2/1 -> Switch/1
  Uniform Random Number1/1 -> Product2/2
  Uniform Random Number/1 -> Product1/2
  Product1/1 -> Add1/2

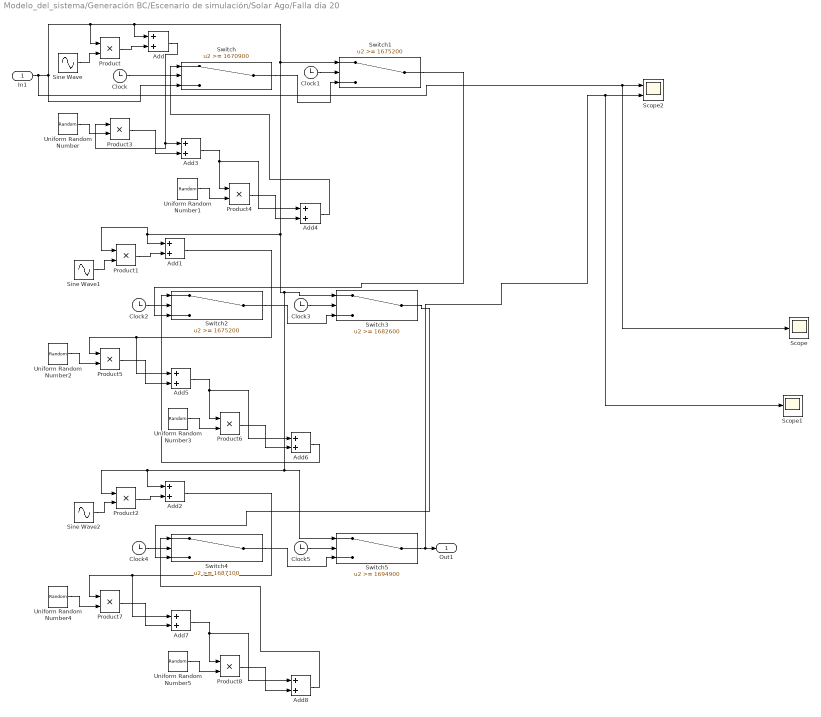
== system Modelo_del_sistema/Generación BC/Escenario de simulación/Solar Ago/Falla día 20 ==
  In1 : Inport
  Add{,1..8} (9 alike) : Sum
  Clock{,1..5} (6 alike) : Clock
  Product{,1..8} (9 alike) : Product
  Scope : Scope
  Scope1 : Scope
  Scope2 : Scope  NumInputPorts=2
  Sine Wave : Sin  Amplitude=0.57  Frequency=1.461206e-3/2  Phase=pi/2-pi/12  SampleTime=0
  Sine Wave1 : Sin  Amplitude=0.92  Frequency=8.49079e-4/2  Phase=pi-pi/2.65  SampleTime=0
  Sine Wave2 : Sin  Amplitude=0.33  Frequency=8.05537e-4/2  Phase=pi-pi/3.4  SampleTime=0
  Switch : Switch  Threshold=1670900
  Switch1 : Switch  Threshold=1675200
  Switch2 : Switch  Threshold=1675200
  Switch3 : Switch  Threshold=1682600
  Switch4 : Switch  Threshold=1687100
  Switch5 : Switch  Threshold=1694900
  Uniform Random Number : UniformRandomNumber  Minimum=-0.5  Maximum=0  Seed=1337  SampleTime=50
  Uniform Random Number1 : UniformRandomNumber  Minimum=-0.25  Maximum=0  Seed=69420  SampleTime=25
  Uniform Random Number2 : UniformRandomNumber  Minimum=-0.5  Maximum=0  Seed=1337  SampleTime=50
  Uniform Random Number3 : UniformRandomNumber  Minimum=-0.25  Maximum=0  Seed=69420  SampleTime=25
  Uniform Random Number4 : UniformRandomNumber  Minimum=-0.5  Maximum=0  Seed=1337  SampleTime=50
  Uniform Random Number5 : UniformRandomNumber  Minimum=-0.25  Maximum=0  Seed=69420  SampleTime=25
  Out1 : Outport
  wires:
  Product/1 -> Add/2
  Clock/1 -> Switch/2
  Sine Wave/1 -> Product/2
  Clock1/1 -> Switch1/2
  Switch/1 -> Switch1/3
  Switch1/1 -> Switch2/3
  Switch2/1 -> Switch3/3
  Clock2/1 -> Switch2/2
  Clock3/1 -> Switch3/2
  Sine Wave1/1 -> Product1/2
  Product1/1 -> Add1/2
  In1/1 -> Scope/1, Scope2/1, Switch/3, Product/1, Add/1, Switch1/1, Product2/1, Add2/1, Switch5/1, Switch3/1, Product1/1, Add1/1
  Switch3/1 -> Switch4/3
  Switch4/1 -> Switch5/3
  Clock4/1 -> Switch4/2
  Clock5/1 -> Switch5/2
  Sine Wave2/1 -> Product2/2
  Product2/1 -> Add2/2
  Switch5/1 -> Out1/1, Scope1/1, Scope2/2
  Add3/1 -> Add4/1, Product4/1
  Add/1 -> Product3/1, Add3/1
  Product4/1 -> Add4/2
  Add4/1 -> Switch/1
  Uniform Random Number1/1 -> Product4/2
  Uniform Random Number/1 -> Product3/2
  Product3/1 -> Add3/2
  Add5/1 -> Add6/1, Product6/1
  Product6/1 -> Add6/2
  Uniform Random Number3/1 -> Product6/2
  Add1/1 -> Add5/1, Product5/1
  Uniform Random Number2/1 -> Product5/2
  Product5/1 -> Add5/2
  Add6/1 -> Switch2/1
  Add7/1 -> Add8/1, Product8/1
  Product8/1 -> Add8/2
  Add8/1 -> Switch4/1
  Uniform Random Number5/1 -> Product8/2
  Add2/1 -> Add7/1, Product7/1
  Uniform Random Number4/1 -> Product7/2
  Product7/1 -> Add7/2

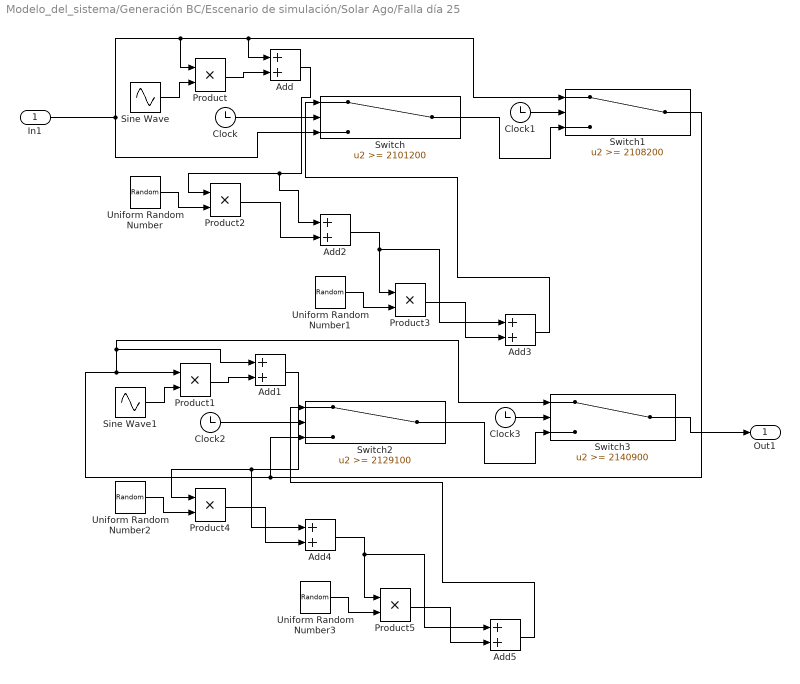
== system Modelo_del_sistema/Generación BC/Escenario de simulación/Solar Ago/Falla día 25 ==
  In1 : Inport
  Add{,1..5} (6 alike) : Sum
  Clock{,1..3} (4 alike) : Clock
  Product{,1..5} (6 alike) : Product
  Sine Wave : Sin  Amplitude=0.62  Frequency=0.000448799  Phase=pi-pi/5.833  SampleTime=0
  Sine Wave1 : Sin  Amplitude=0.66  Frequency=0.000266237  Phase=pi/2+pi/14.798  SampleTime=0
  Switch : Switch  Threshold=2101200
  Switch1 : Switch  Threshold=2108200
  Switch2 : Switch  Threshold=2129100
  Switch3 : Switch  Threshold=2140900
  Uniform Random Number : UniformRandomNumber  Minimum=-0.5  Maximum=0  Seed=1337  SampleTime=50
  Uniform Random Number1 : UniformRandomNumber  Minimum=-0.25  Maximum=0  Seed=69420  SampleTime=25
  Uniform Random Number2 : UniformRandomNumber  Minimum=-0.5  Maximum=0  Seed=1337  SampleTime=50
  Uniform Random Number3 : UniformRandomNumber  Minimum=-0.25  Maximum=0  Seed=69420  SampleTime=25
  Out1 : Outport
  wires:
  Switch3/1 -> Out1/1
  Product/1 -> Add/2
  Clock/1 -> Switch/2
  Sine Wave/1 -> Product/2
  Clock1/1 -> Switch1/2
  Switch/1 -> Switch1/3
  In1/1 -> Switch/3, Product/1, Add/1, Switch1/1
  Product1/1 -> Add1/2
  Clock2/1 -> Switch2/2
  Sine Wave1/1 -> Product1/2
  Clock3/1 -> Switch3/2
  Switch2/1 -> Switch3/3
  Switch1/1 -> Switch3/1, Add1/1, Product1/1, Switch2/3
  Add2/1 -> Add3/1, Product3/1
  Add/1 -> Add2/1, Product2/1
  Product3/1 -> Add3/2
  Add3/1 -> Switch/1
  Uniform Random Number1/1 -> Product3/2
  Uniform Random Number/1 -> Product2/2
  Product2/1 -> Add2/2
  Add4/1 -> Add5/1, Product5/1
  Product5/1 -> Add5/2
  Add5/1 -> Switch2/1
  Uniform Random Number3/1 -> Product5/2
  Add1/1 -> Add4/1, Product4/1
  Uniform Random Number2/1 -> Product4/2
  Product4/1 -> Add4/2

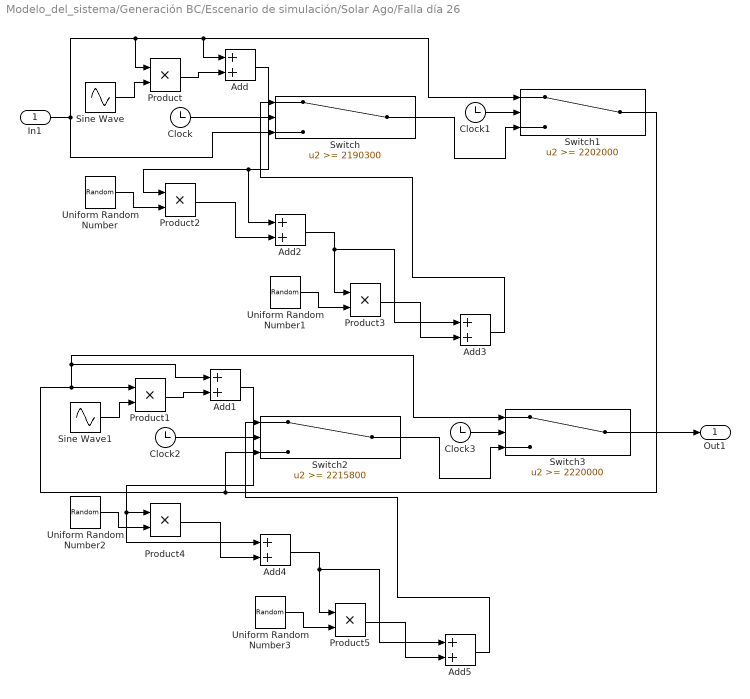
== system Modelo_del_sistema/Generación BC/Escenario de simulación/Solar Ago/Falla día 26 ==
  In1 : Inport
  Add{,1..5} (6 alike) : Sum
  Clock{,1..3} (4 alike) : Clock
  Product{,1..5} (6 alike) : Product
  Sine Wave : Sin  Amplitude=0.79  Frequency=0.000268512  Phase=-pi/4+pi/22.21  SampleTime=0
  Sine Wave1 : Sin  Amplitude=0.39  Frequency=0.000747998  Phase=-pi/2-pi/14.04  SampleTime=0
  Switch : Switch  Threshold=2190300
  Switch1 : Switch  Threshold=2202000
  Switch2 : Switch  Threshold=2215800
  Switch3 : Switch  Threshold=2220000
  Uniform Random Number : UniformRandomNumber  Minimum=-0.5  Maximum=0  Seed=1337  SampleTime=50
  Uniform Random Number1 : UniformRandomNumber  Minimum=-0.25  Maximum=0  Seed=69420  SampleTime=25
  Uniform Random Number2 : UniformRandomNumber  Minimum=-0.5  Maximum=0  Seed=1337  SampleTime=50
  Uniform Random Number3 : UniformRandomNumber  Minimum=-0.25  Maximum=0  Seed=69420  SampleTime=25
  Out1 : Outport
  wires:
  Product/1 -> Add/2
  Clock/1 -> Switch/2
  Sine Wave/1 -> Product/2
  Clock1/1 -> Switch1/2
  Switch/1 -> Switch1/3
  In1/1 -> Switch/3, Product/1, Add/1, Switch1/1
  Product1/1 -> Add1/2
  Clock2/1 -> Switch2/2
  Sine Wave1/1 -> Product1/2
  Clock3/1 -> Switch3/2
  Switch2/1 -> Switch3/3
  Switch3/1 -> Out1/1
  Switch1/1 -> Switch3/1, Add1/1, Product1/1, Switch2/3
  Add2/1 -> Add3/1, Product3/1
  Product3/1 -> Add3/2
  Add3/1 -> Switch/1
  Uniform Random Number1/1 -> Product3/2
  Add/1 -> Add2/1, Product2/1
  Uniform Random Number/1 -> Product2/2
  Product2/1 -> Add2/2
  Add4/1 -> Add5/1, Product5/1
  Product5/1 -> Add5/2
  Add5/1 -> Switch2/1
  Uniform Random Number3/1 -> Product5/2
  Add1/1 -> Add4/1, Product4/1
  Uniform Random Number2/1 -> Product4/2
  Product4/1 -> Add4/2

== system Modelo_del_sistema/Generación BC/Escenario de simulación/Solar Ago/Falla día 28 ==
  In1 : Inport
  Add : Sum
  Add1 : Sum
  Add2 : Sum
  Clock : Clock
  Clock1 : Clock
  Product : Product
  Product1 : Product
  Product2 : Product
  Sine Wave : Sin  Amplitude=0.56  Frequency=2.596358e-3/2  Phase=pi/7.15  SampleTime=0
  Switch : Switch  Threshold=2378520
  Switch1 : Switch  Threshold=2380940
  Uniform Random Number : UniformRandomNumber  Minimum=-0.5  Maximum=0  Seed=1337  SampleTime=50
  Uniform Random Number1 : UniformRandomNumber  Minimum=-0.25  Maximum=0  Seed=69420  SampleTime=25
  Out1 : Outport
  wires:
  Product/1 -> Add/2
  Clock/1 -> Switch/2
  In1/1 -> Switch/3, Product/1, Add/1, Switch1/1
  Switch1/1 -> Out1/1
  Sine Wave/1 -> Product/2
  Clock1/1 -> Switch1/2
  Switch/1 -> Switch1/3
  Add1/1 -> Add2/1, Product2/1
  Product2/1 -> Add2/2
  Add2/1 -> Switch/1
  Uniform Random Number1/1 -> Product2/2
  Add/1 -> Add1/1, Product1/1
  Uniform Random Number/1 -> Product1/2
  Product1/1 -> Add1/2

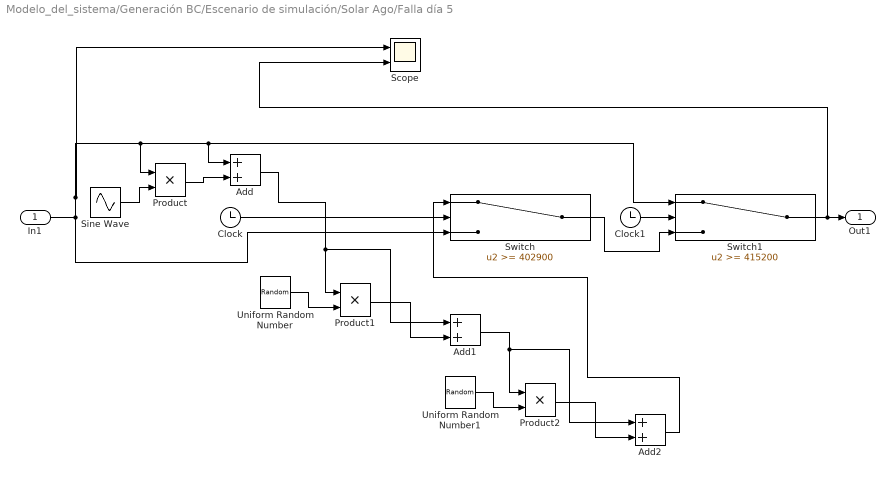
== system Modelo_del_sistema/Generación BC/Escenario de simulación/Solar Ago/Falla día 5 ==
  In1 : Inport
  Add : Sum
  Add1 : Sum
  Add2 : Sum
  Clock : Clock
  Clock1 : Clock
  Product : Product
  Product1 : Product
  Product2 : Product
  Scope : Scope  NumInputPorts=2
  Sine Wave : Sin  Amplitude=0.81  Frequency=0.000255414  Phase=pi/4-pi/165  SampleTime=0
  Switch : Switch  Threshold=402900
  Switch1 : Switch  Threshold=415200
  Uniform Random Number : UniformRandomNumber  Minimum=-0.5  Maximum=0  Seed=1337  SampleTime=50
  Uniform Random Number1 : UniformRandomNumber  Minimum=-0.25  Maximum=0  Seed=69420  SampleTime=25
  Out1 : Outport
  wires:
  Add/1 -> Add1/1, Product1/1
  Product/1 -> Add/2
  Clock/1 -> Switch/2
  Switch1/1 -> Scope/2, Out1/1
  Sine Wave/1 -> Product/2
  Clock1/1 -> Switch1/2
  Switch/1 -> Switch1/3
  In1/1 -> Switch/3, Scope/1, Product/1, Add/1, Switch1/1
  Uniform Random Number/1 -> Product1/2
  Product1/1 -> Add1/2
  Add2/1 -> Switch/1
  Add1/1 -> Add2/1, Product2/1
  Uniform Random Number1/1 -> Product2/2
  Product2/1 -> Add2/2

== system Modelo_del_sistema/Generación BC/Escenario de simulación/Solar Ago/Falla día 9 ==
  In1 : Inport
  Add : Sum
  Add1 : Sum
  Add2 : Sum
  Clock : Clock
  Clock1 : Clock
  Product : Product
  Product1 : Product
  Product2 : Product
  Sine Wave : Sin  Amplitude=0.56  Frequency=0.000171672  Phase=pi+pi/5.9052  SampleTime=0
  Switch : Switch  Threshold=728900
  Switch1 : Switch  Threshold=747200
  Uniform Random Number : UniformRandomNumber  Minimum=-0.5  Maximum=0  Seed=1337  SampleTime=50
  Uniform Random Number1 : UniformRandomNumber  Minimum=-0.25  Maximum=0  Seed=69420  SampleTime=25
  Out1 : Outport
  wires:
  Product/1 -> Add/2
  Clock/1 -> Switch/2
  Sine Wave/1 -> Product/2
  Clock1/1 -> Switch1/2
  Switch/1 -> Switch1/3
  In1/1 -> Switch/3, Product/1, Add/1, Switch1/1
  Switch1/1 -> Out1/1
  Add1/1 -> Add2/1, Product2/1
  Product2/1 -> Add2/2
  Add2/1 -> Switch/1
  Uniform Random Number1/1 -> Product2/2
  Add/1 -> Add1/1, Product1/1
  Uniform Random Number/1 -> Product1/2
  Product1/1 -> Add1/2

== system Modelo_del_sistema/Generación BC/Escenario de simulación/Solar Dic/Falla día 13 ==
  In1 : Inport
  Add : Sum
  Add1 : Sum
  Add2 : Sum
  Clock : Clock
  Clock1 : Clock
  Product : Product
  Product1 : Product
  Product2 : Product
  Sine Wave : Sin  Amplitude=0.31  Frequency=0.000184800  Phase=pi/34  SampleTime=0
  Switch : Switch  Threshold=1070500
  Switch1 : Switch  Threshold=1087500
  Uniform Random Number : UniformRandomNumber  Minimum=-0.5  Maximum=0  Seed=1337  SampleTime=50
  Uniform Random Number1 : UniformRandomNumber  Minimum=-0.25  Maximum=0  Seed=69420  SampleTime=25
  Out1 : Outport
  wires:
  Product/1 -> Add/2
  Clock/1 -> Switch/2
  In1/1 -> Switch/3, Product/1, Add/1, Switch1/1
  Switch1/1 -> Out1/1
  Sine Wave/1 -> Product/2
  Clock1/1 -> Switch1/2
  Switch/1 -> Switch1/3
  Add1/1 -> Add2/1, Product2/1
  Product2/1 -> Add2/2
  Add2/1 -> Switch/1
  Uniform Random Number1/1 -> Product2/2
  Add/1 -> Add1/1, Product1/1
  Uniform Random Number/1 -> Product1/2
  Product1/1 -> Add1/2

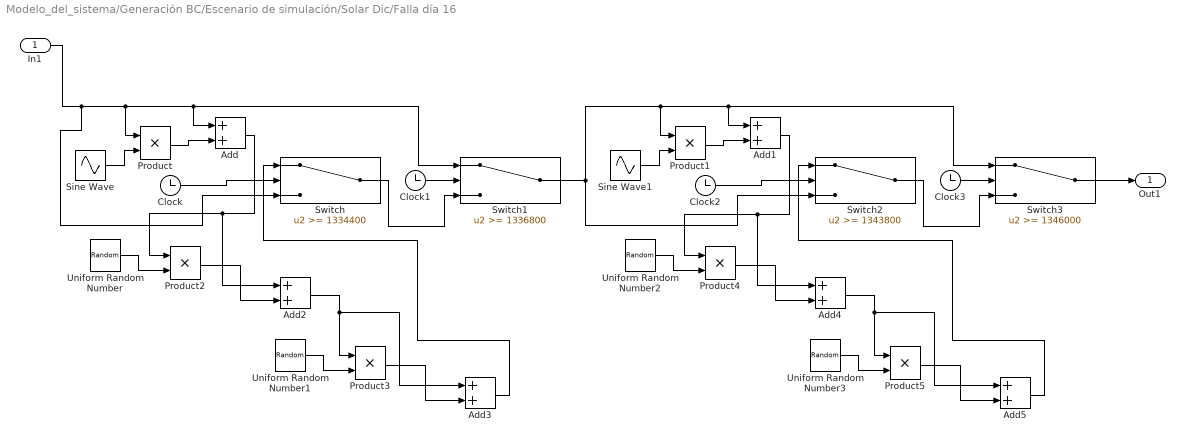
== system Modelo_del_sistema/Generación BC/Escenario de simulación/Solar Dic/Falla día 16 ==
  In1 : Inport
  Add{,1..5} (6 alike) : Sum
  Clock{,1..3} (4 alike) : Clock
  Product{,1..5} (6 alike) : Product
  Sine Wave : Sin  Amplitude=0.57  Frequency=0.001308997  Phase=pi  SampleTime=0
  Sine Wave1 : Sin  Amplitude=0.76  Frequency=0.001427997  Phase=pi/5.5  SampleTime=0
  Switch : Switch  Threshold=1334400
  Switch1 : Switch  Threshold=1336800
  Switch2 : Switch  Threshold=1343800
  Switch3 : Switch  Threshold=1346000
  Uniform Random Number : UniformRandomNumber  Minimum=-0.5  Maximum=0  Seed=1337  SampleTime=50
  Uniform Random Number1 : UniformRandomNumber  Minimum=-0.25  Maximum=0  Seed=69420  SampleTime=25
  Uniform Random Number2 : UniformRandomNumber  Minimum=-0.5  Maximum=0  Seed=1337  SampleTime=50
  Uniform Random Number3 : UniformRandomNumber  Minimum=-0.25  Maximum=0  Seed=69420  SampleTime=25
  Out1 : Outport
  wires:
  Product/1 -> Add/2
  Clock/1 -> Switch/2
  In1/1 -> Switch/3, Product/1, Add/1, Switch1/1
  Sine Wave/1 -> Product/2
  Clock1/1 -> Switch1/2
  Switch/1 -> Switch1/3
  Product1/1 -> Add1/2
  Clock2/1 -> Switch2/2
  Switch1/1 -> Product1/1, Add1/1, Switch3/1, Switch2/3
  Sine Wave1/1 -> Product1/2
  Clock3/1 -> Switch3/2
  Switch2/1 -> Switch3/3
  Switch3/1 -> Out1/1
  Add2/1 -> Add3/1, Product3/1
  Product3/1 -> Add3/2
  Add3/1 -> Switch/1
  Uniform Random Number1/1 -> Product3/2
  Add/1 -> Add2/1, Product2/1
  Uniform Random Number/1 -> Product2/2
  Product2/1 -> Add2/2
  Add4/1 -> Add5/1, Product5/1
  Product5/1 -> Add5/2
  Add5/1 -> Switch2/1
  Uniform Random Number3/1 -> Product5/2
  Add1/1 -> Add4/1, Product4/1
  Uniform Random Number2/1 -> Product4/2
  Product4/1 -> Add4/2

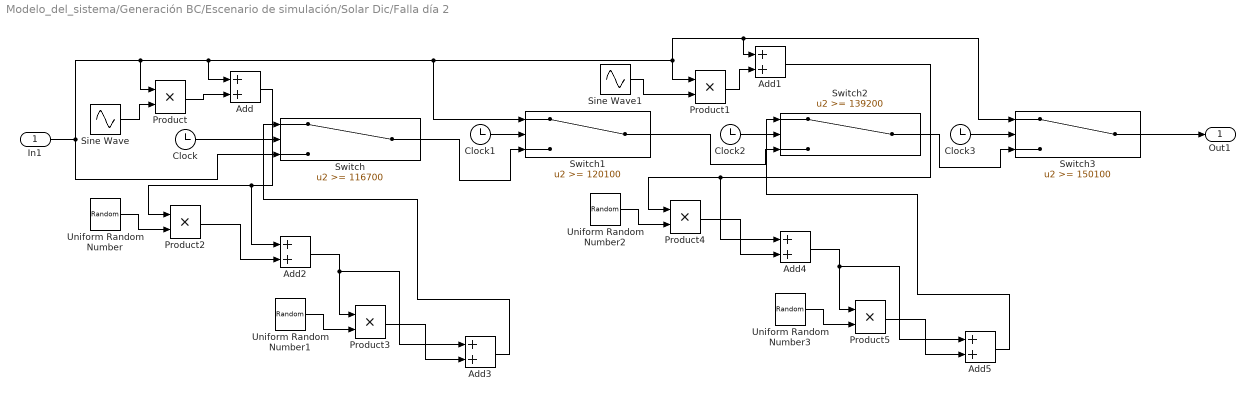
== system Modelo_del_sistema/Generación BC/Escenario de simulación/Solar Dic/Falla día 2 ==
  In1 : Inport
  Add{,1..5} (6 alike) : Sum
  Clock{,1..3} (4 alike) : Clock
  Product{,1..5} (6 alike) : Product
  Sine Wave : Sin  Amplitude=0.63  Frequency=9.23998e-4  Phase=2*pi/4+pi/5.7  SampleTime=0
  Sine Wave1 : Sin  Amplitude=0.82  Frequency=2.88220e-4  Phase=pi/4.36  SampleTime=0
  Switch : Switch  Threshold=116700
  Switch1 : Switch  Threshold=120100
  Switch2 : Switch  Threshold=139200
  Switch3 : Switch  Threshold=150100
  Uniform Random Number : UniformRandomNumber  Minimum=-0.5  Maximum=0  Seed=1337  SampleTime=50
  Uniform Random Number1 : UniformRandomNumber  Minimum=-0.25  Maximum=0  Seed=69420  SampleTime=25
  Uniform Random Number2 : UniformRandomNumber  Minimum=-0.5  Maximum=0  Seed=1337  SampleTime=50
  Uniform Random Number3 : UniformRandomNumber  Minimum=-0.25  Maximum=0  Seed=69420  SampleTime=25
  Out1 : Outport
  wires:
  Product/1 -> Add/2
  Clock/1 -> Switch/2
  Clock1/1 -> Switch1/2
  Switch/1 -> Switch1/3
  Switch1/1 -> Switch2/3
  Switch2/1 -> Switch3/3
  Clock2/1 -> Switch2/2
  Clock3/1 -> Switch3/2
  Sine Wave1/1 -> Product1/2
  Product1/1 -> Add1/2
  In1/1 -> Switch/3, Product/1, Add/1, Switch1/1, Add1/1, Switch3/1, Product1/1
  Sine Wave/1 -> Product/2
  Switch3/1 -> Out1/1
  Add2/1 -> Add3/1, Product3/1
  Product3/1 -> Add3/2
  Uniform Random Number1/1 -> Product3/2
  Add/1 -> Add2/1, Product2/1
  Uniform Random Number/1 -> Product2/2
  Product2/1 -> Add2/2
  Add3/1 -> Switch/1
  Add4/1 -> Add5/1, Product5/1
  Product5/1 -> Add5/2
  Add5/1 -> Switch2/1
  Uniform Random Number3/1 -> Product5/2
  Add1/1 -> Add4/1, Product4/1
  Uniform Random Number2/1 -> Product4/2
  Product4/1 -> Add4/2

== system Modelo_del_sistema/Generación BC/Escenario de simulación/Solar Dic/Falla día 21 ==
  In1 : Inport
  Add : Sum
  Add1 : Sum
  Add2 : Sum
  Clock : Clock
  Clock1 : Clock
  Product : Product
  Product1 : Product
  Product2 : Product
  Sine Wave : Sin  Amplitude=0.43  Frequency=0.000193925  Phase=pi/4+pi/2-pi/111  SampleTime=0
  Switch : Switch  Threshold=1753800
  Switch1 : Switch  Threshold=1770000
  Uniform Random Number : UniformRandomNumber  Minimum=-0.5  Maximum=0  Seed=1337  SampleTime=50
  Uniform Random Number1 : UniformRandomNumber  Minimum=-0.25  Maximum=0  Seed=69420  SampleTime=25
  Out1 : Outport
  wires:
  Product/1 -> Add/2
  Clock/1 -> Switch/2
  In1/1 -> Switch/3, Product/1, Add/1, Switch1/1
  Switch1/1 -> Out1/1
  Sine Wave/1 -> Product/2
  Clock1/1 -> Switch1/2
  Switch/1 -> Switch1/3
  Add1/1 -> Add2/1, Product2/1
  Product2/1 -> Add2/2
  Add2/1 -> Switch/1
  Uniform Random Number1/1 -> Product2/2
  Add/1 -> Add1/1, Product1/1
  Uniform Random Number/1 -> Product1/2
  Product1/1 -> Add1/2

== system Modelo_del_sistema/Generación BC/Escenario de simulación/Solar Dic/Falla día 23 ==
  In1 : Inport
  Add : Sum
  Add1 : Sum
  Add2 : Sum
  Clock : Clock
  Clock1 : Clock
  Product : Product
  Product1 : Product
  Product2 : Product
  Sine Wave : Sin  Amplitude=0.88  Frequency=0.000263999  Phase=-pi/8-pi/3.045  SampleTime=0
  Switch : Switch  Threshold=1945100
  Switch1 : Switch  Threshold=1957000
  Uniform Random Number : UniformRandomNumber  Minimum=-0.5  Maximum=0  Seed=1337  SampleTime=50
  Uniform Random Number1 : UniformRandomNumber  Minimum=-0.25  Maximum=0  Seed=69420  SampleTime=25
  Out1 : Outport
  wires:
  Product/1 -> Add/2
  Clock/1 -> Switch/2
  In1/1 -> Switch/3, Product/1, Add/1, Switch1/1
  Switch1/1 -> Out1/1
  Sine Wave/1 -> Product/2
  Clock1/1 -> Switch1/2
  Switch/1 -> Switch1/3
  Add1/1 -> Add2/1, Product2/1
  Product2/1 -> Add2/2
  Add2/1 -> Switch/1
  Uniform Random Number1/1 -> Product2/2
  Add/1 -> Add1/1, Product1/1
  Uniform Random Number/1 -> Product1/2
  Product1/1 -> Add1/2
